simulink model "grid_connected_inverter_model"  (R2021a)
settings: Solver=VariableStepAuto  StartTime=0.0  StopTime=0.2  RelTol=1e-3
values from neighbouring files (symbols this model uses):
  I = 0    [grid_connected_inverter_tuning.m]
  I_max = A_inv/V_dc    (= 72.4637681159)    [grid_connected_inverter_tuning.m]
  Ki_current = alpha_current*R    [grid_connected_inverter_tuning.m]
  Ki_DC_voltage = Kp_DC_voltage/Ti_DC_voltage    [grid_connected_inverter_tuning.m]
  Ki_PLL = Kp_PLL/Ti_PLL    (= 21.16)    [grid_connected_inverter_tuning.m]
  Kp_current = alpha_current*L    [grid_connected_inverter_tuning.m]
  Kp_DC_voltage = 1    [grid_connected_inverter_tuning.m]
  Kp_PLL = 9.2/settling_time    (= 9.2)    [grid_connected_inverter_tuning.m]
  L = 1e-3    (= 0.001)    [grid_connected_inverter_tuning.m]
  omega = 2*pi*50    (= 314.159265359)    [grid_connected_inverter_tuning.m]
  R = 0.314    [grid_connected_inverter_tuning.m]
  sampling_time = 1/(2*switching_frequency)    (= 0.0002)    [grid_connected_inverter_tuning.m]
  V_a = 400    [grid_connected_inverter_tuning.m]
  V_b = 400    [grid_connected_inverter_tuning.m]
  V_c = 400    [grid_connected_inverter_tuning.m]
  V_dc = 690    [grid_connected_inverter_tuning.m]
libraries: fl_lib x17, ee_lib x15, nesl_utility x15, spsAlphaBetaZerotodq0Lib x6, pid_lib x5, spsabctoAlphaBetaZeroLib x4, spsAlphaBetaZerotoabcLib x1, spsdq0toAlphaBetaZeroLib x1, spsPWMGenerator2LevelLib x1
settings Model: SimulationMode=accelerator  Creator=giuli  LastModifiedBy=giuli
settings ModelReferenceCC: ModelReferenceMinAlgLoopOccurrences=on

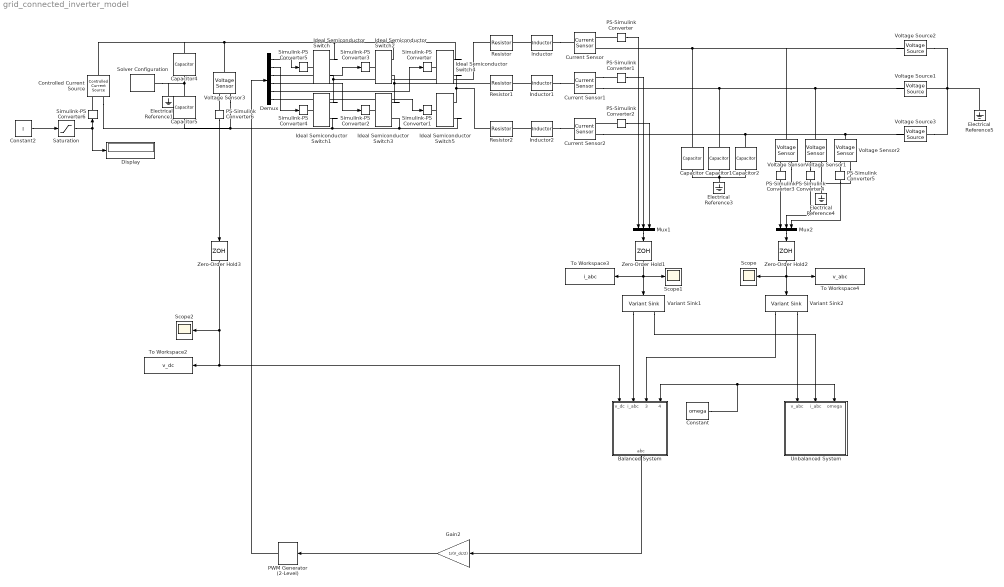
== system grid_connected_inverter_model ==
  Balanced System : Subsystem
  Capacitor : fl_lib/Electrical/Electrical Elements/Capacitor  c=C F  r=1e-6 Ohm  g=0 1/Ohm  i_specify=off  i_priority=None  i=0 A  i_nominal_specify=off  i_nominal_unit=A  i_nominal_value=1  v_specify=off  v_priority=None  v=0 V  v_nominal_specify=off  v_nominal_unit=V  v_nominal_value=1  vc_specify=off  vc_priority=High  vc=0 V  vc_nominal_specify=off  vc_nominal_unit=V  vc_nominal_value=1
  Capacitor1 : fl_lib/Electrical/Electrical Elements/Capacitor  c=C F  r=1e-6 Ohm  g=0 1/Ohm  i_specify=off  i_priority=None  i=0 A  i_nominal_specify=off  i_nominal_unit=A  i_nominal_value=1  v_specify=off  v_priority=None  v=0 V  v_nominal_specify=off  v_nominal_unit=V  v_nominal_value=1  vc_specify=off  vc_priority=High  vc=0 V  vc_nominal_specify=off  vc_nominal_unit=V  vc_nominal_value=1
  Capacitor2 : fl_lib/Electrical/Electrical Elements/Capacitor  c=C F  r=1e-6 Ohm  g=0 1/Ohm  i_specify=off  i_priority=None  i=0 A  i_nominal_specify=off  i_nominal_unit=A  i_nominal_value=1  v_specify=off  v_priority=None  v=0 V  v_nominal_specify=off  v_nominal_unit=V  v_nominal_value=1  vc_specify=off  vc_priority=High  vc=0 V  vc_nominal_specify=off  vc_nominal_unit=V  vc_nominal_value=1
  Capacitor4 : fl_lib/Electrical/Electrical Elements/Capacitor  c=C_dc F  r=1e-6 Ohm  g=0 1/Ohm  i_specify=off  i_priority=High  i=0 A  i_nominal_specify=off  i_nominal_unit=A  i_nominal_value=1  v_specify=off  v_priority=High  v=V_dc/2 V  v_nominal_specify=off  v_nominal_unit=V  v_nominal_value=1  vc_specify=on  vc_priority=High  vc=V_dc/2 V  vc_nominal_specify=off  vc_nominal_unit=V  vc_nominal_value=1
  Capacitor5 : fl_lib/Electrical/Electrical Elements/Capacitor  c=C_dc F  r=1e-6 Ohm  g=0 1/Ohm  i_specify=off  i_priority=High  i=0 A  i_nominal_specify=off  i_nominal_unit=A  i_nominal_value=1  v_specify=off  v_priority=High  v=V_dc/2 V  v_nominal_specify=off  v_nominal_unit=V  v_nominal_value=1  vc_specify=on  vc_priority=High  vc=V_dc/2 V  vc_nominal_specify=off  vc_nominal_unit=V  vc_nominal_value=1
  Constant : Constant  Value=omega
  Constant2 : Constant  Value=I
  Controlled Current Source : fl_lib/Electrical/Electrical Sources/Controlled Current Source
  Current Sensor : fl_lib/Electrical/Electrical Sensors/Current Sensor
  Current Sensor1 : fl_lib/Electrical/Electrical Sensors/Current Sensor
  Current Sensor2 : fl_lib/Electrical/Electrical Sensors/Current Sensor
  Demux : Demux  Outputs=6
  Display : Display
  Electrical Reference{1,3..5} (4 alike) : fl_lib/Electrical/Electrical Elements/Electrical Reference
  Gain2 : Gain  Gain=1/(V_dc/2)
  Ideal Semiconductor Switch{,1..5} (6 alike) : ee_lib/Semiconductors & Converters/Ideal Semiconductor Switch  Ron=0.001 Ohm  Goff=1e-6 1/Ohm  Vth=0.5 V  diode_param=1  diode_Vf=0.8 V  diode_Ron=0.001 Ohm  diode_Goff=1e-5 1/Ohm  diode_C=50e-9 F  diode_iRM=-235 A  diode_iF=300 A  diode_idot=-50 A/us  diode_trr_param=1  diode_trr_factor=3  diode_trr=15 us  diode_Qrr=1500 s*uA
      settings: SourceProductBaseCode=PS
  Inductor : ee_lib/Passive/Inductor  l=L H  L_tol=20  enable_L_tol=0  tol_distribution=1  nSigma=4  r=0 Ohm  g=1e-9 1/Ohm  enable_operating_limits=0  operating_limit_action=2  max_working_current=1 A  power_rating=1 W  enable_faults=0  fault_action=1  lambdaPercent=50  k_faulted=0.9999  turnsShort=0  openCct=0  groundShort=0  groundShortG=0 1/Ohm  tau_fault=1e-3 s  enable_temporal_fault=0  t_fault=1 s  enable_behavioral_fault=0  max_permissible_voltage=100 V  n_fail_on_voltage=1  max_permissible_current=1 A  t_fail_on_current=1 s  i_L_specify=off  i_L_priority=High  i_L=0 A  i_L_nominal_specify=off  i_L_nominal_unit=A  i_L_nominal_value=1
  Inductor1 : ee_lib/Passive/Inductor  l=L H  L_tol=20  enable_L_tol=0  tol_distribution=1  nSigma=4  r=0 Ohm  g=1e-9 1/Ohm  enable_operating_limits=0  operating_limit_action=2  max_working_current=1 A  power_rating=1 W  enable_faults=0  fault_action=1  lambdaPercent=50  k_faulted=0.9999  turnsShort=0  openCct=0  groundShort=0  groundShortG=0 1/Ohm  tau_fault=1e-3 s  enable_temporal_fault=0  t_fault=1 s  enable_behavioral_fault=0  max_permissible_voltage=100 V  n_fail_on_voltage=1  max_permissible_current=1 A  t_fail_on_current=1 s  i_L_specify=off  i_L_priority=High  i_L=0 A  i_L_nominal_specify=off  i_L_nominal_unit=A  i_L_nominal_value=1
  Inductor2 : ee_lib/Passive/Inductor  l=L H  L_tol=20  enable_L_tol=0  tol_distribution=1  nSigma=4  r=0 Ohm  g=1e-9 1/Ohm  enable_operating_limits=0  operating_limit_action=2  max_working_current=1 A  power_rating=1 W  enable_faults=0  fault_action=1  lambdaPercent=50  k_faulted=0.9999  turnsShort=0  openCct=0  groundShort=0  groundShortG=0 1/Ohm  tau_fault=1e-3 s  enable_temporal_fault=0  t_fault=1 s  enable_behavioral_fault=0  max_permissible_voltage=100 V  n_fail_on_voltage=1  max_permissible_current=1 A  t_fail_on_current=1 s  i_L_specify=off  i_L_priority=High  i_L=0 A  i_L_nominal_specify=off  i_L_nominal_unit=A  i_L_nominal_value=1
  Mux1 : Mux  Inputs=3
  Mux2 : Mux  Inputs=3
  PS-Simulink Converter{,1..6} (7 alike) : nesl_utility/PS-Simulink Converter  PhysicalDomain=network_engine_domain  SubClassName=ps_output  LeftPortType=input  RightPortType=output  PseudoPeriodic=off  Frequencies=[]  Unit=inherit  AffineConversion=off
      settings: SourceProductBaseCode=PW,SS
  PWM Generator (2-Level) : spsPWMGenerator2LevelLib/PWM Generator (2-Level)  ModulatorType=Three-phase bridge (6 pulses)  ModulatorMode=Unsynchronized  Fc=switching_frequency  Pc=0  nF=27  MinMax="[ -1  1 ]"  SamplingTechnique=Asymmetrical regular (double edge)  ModulatingSignals=off  m=0.8  Freq=60  Phase=0  Ts=1e-6  ShowCarrierOutport=off
  Resistor : ee_lib/Passive/Resistor  R=R Ohm  R_tol=5  enable_R_tol=0  tol_distribution=1  nSigma=4  enable_operating_limits=0  operating_limit_action=2  max_working_voltage=100 V  power_rating=1 W  enable_faults=0  fault_action=1  R_faulted=inf Ohm  enable_temporal_fault=0  t_fault=1 s  enable_behavioral_fault=0  max_permissible_current=1 A  t_fail_on_current=1 s  noise_mode=0  sample_time=1e-3 s  repeatability=1  auto_seed=3499211588  user_seed=0  Tdevice=25 degC  alpha=3.93e-3 1/K  Tmeas=25 degC  thermal_mass=100 J/K  power_derating_T1=70 degC  power_derating_T2=155 degC  operating_temperature_range_vec=[-50, 150] degC  temperature_specify=off  temperature_priority=High  temperature=298.15 K  temperature_nominal_specify=off  temperature_nominal_unit=K  temperature_nominal_value=1
  Resistor1 : ee_lib/Passive/Resistor  R=R Ohm  R_tol=5  enable_R_tol=0  tol_distribution=1  nSigma=4  enable_operating_limits=0  operating_limit_action=2  max_working_voltage=100 V  power_rating=1 W  enable_faults=0  fault_action=1  R_faulted=inf Ohm  enable_temporal_fault=0  t_fault=1 s  enable_behavioral_fault=0  max_permissible_current=1 A  t_fail_on_current=1 s  noise_mode=0  sample_time=1e-3 s  repeatability=1  auto_seed=3890346746  user_seed=0  Tdevice=25 degC  alpha=3.93e-3 1/K  Tmeas=25 degC  thermal_mass=100 J/K  power_derating_T1=70 degC  power_derating_T2=155 degC  operating_temperature_range_vec=[-50, 150] degC  temperature_specify=off  temperature_priority=High  temperature=298.15 K  temperature_nominal_specify=off  temperature_nominal_unit=K  temperature_nominal_value=1
  Resistor2 : ee_lib/Passive/Resistor  R=R Ohm  R_tol=5  enable_R_tol=0  tol_distribution=1  nSigma=4  enable_operating_limits=0  operating_limit_action=2  max_working_voltage=100 V  power_rating=1 W  enable_faults=0  fault_action=1  R_faulted=inf Ohm  enable_temporal_fault=0  t_fault=1 s  enable_behavioral_fault=0  max_permissible_current=1 A  t_fail_on_current=1 s  noise_mode=0  sample_time=1e-3 s  repeatability=1  auto_seed=545404223  user_seed=0  Tdevice=25 degC  alpha=3.93e-3 1/K  Tmeas=25 degC  thermal_mass=100 J/K  power_derating_T1=70 degC  power_derating_T2=155 degC  operating_temperature_range_vec=[-50, 150] degC  temperature_specify=off  temperature_priority=High  temperature=298.15 K  temperature_nominal_specify=off  temperature_nominal_unit=K  temperature_nominal_value=1
  Saturation : Saturate  UpperLimit=I_max  LowerLimit=0
  Scope : Scope
  Scope1 : Scope
  Scope2 : Scope
  Simulink-PS Converter{,1..6} (7 alike) : nesl_utility/Simulink-PS Converter  PhysicalDomain=network_engine_domain  SubClassName=ps_input  LeftPortType=input  RightPortType=output  PseudoPeriodic=off  Frequencies=[]  NoiseDistribution=none  NoiseParameters=[]  Unit=1  AffineConversion=off  FilteringAndDerivatives=provide  SimscapeFilterOrder=1  InputFilterTimeConstant=0.001  UdotUserProvided=0
      settings: SourceProductBaseCode=PW,SS
  Solver Configuration : nesl_utility/Solver Configuration  PhysicalDomain=network_engine_domain  SubClassName=solver  LeftPortType=input  RightPortType=generic  Tones=[]  Harmonics=[]  SimulateNoise=off  Profile=off  UseLocalSampling=off  EnableSwitchedLinearOptims=on  FrequencyDomain=off  UseCCode=off  RelTol=0.001  AbsTol=1e-06  MinStep=1e-09  ToWorkspace=off  RevertToSquareIcSolve=off  NumHomotopyIterations=100  PhasorMode=off  PhasorModeNumHarmonics=1  DoDC=off  ResidualTolerance=1e-09  UseLocalSolver=off  LocalSolverChoice=NE_BACKWARD_EULER_ADVANCER  LocalSolverSampleTime=0.001  DoFixedCost=off  MaxNonlinIter=3  MaxModeIter=2  ComputeImpulses=off  ImpulseIterations=2  LinearAlgebra=auto  EquationFormulation=NE_TIME_EF  DelaysMemoryBudget=1024  AutomaticFiltering=on  FilteringTimeConstant=0.001  PartitionStorageMethod=AS_NEEDED  PartitionMemoryBudget=1024  PartitionMethod=ROBUST
      settings: SourceProductBaseCode=PW,SS
  To Workspace2 : ToWorkspace  VariableName=v_dc  SaveFormat=Timeseries  SampleTime=-1
  To Workspace3 : ToWorkspace  VariableName=i_abc  SaveFormat=Timeseries  SampleTime=-1
  To Workspace4 : ToWorkspace  VariableName=v_abc  SaveFormat=Timeseries  SampleTime=-1
  Unbalanced System : Subsystem
  Variant Sink1 : VariantSink
  Variant Sink2 : VariantSink
  Voltage Sensor{,1..3} (4 alike) : fl_lib/Electrical/Electrical Sensors/Voltage Sensor
  Voltage Source1 : ee_lib/Sources/Voltage Source  dc_voltage=0 V  ac_voltage=V_b*sqrt(2)/sqrt(3) V  ac_shift=phi_b rad  ac_frequency=50 Hz  noise_mode=0  PSD=0 V^2/Hz  repeatability=1  auto_seed=1127352614  user_seed=0  sample_time=1e-3 s  i_specify=off  i_priority=None  i=0 A  i_nominal_specify=off  i_nominal_unit=A  i_nominal_value=1  v_specify=off  v_priority=None  v=0 V  v_nominal_specify=off  v_nominal_unit=V  v_nominal_value=1
  Voltage Source2 : ee_lib/Sources/Voltage Source  dc_voltage=0 V  ac_voltage=V_a*sqrt(2)/sqrt(3) V  ac_shift=phi_a rad  ac_frequency=50 Hz  noise_mode=0  PSD=0 V^2/Hz  repeatability=1  auto_seed=3440331608  user_seed=0  sample_time=1e-3 s  i_specify=off  i_priority=None  i=0 A  i_nominal_specify=off  i_nominal_unit=A  i_nominal_value=1  v_specify=off  v_priority=None  v=0 V  v_nominal_specify=off  v_nominal_unit=V  v_nominal_value=1
  Voltage Source3 : ee_lib/Sources/Voltage Source  dc_voltage=0 V  ac_voltage=V_c*sqrt(2)/sqrt(3) V  ac_shift=phi_c rad  ac_frequency=50 Hz  noise_mode=0  PSD=0 V^2/Hz  repeatability=1  auto_seed=830791639  user_seed=0  sample_time=1e-3 s  i_specify=off  i_priority=None  i=0 A  i_nominal_specify=off  i_nominal_unit=A  i_nominal_value=1  v_specify=off  v_priority=None  v=0 V  v_nominal_specify=off  v_nominal_unit=V  v_nominal_value=1
  Zero-Order Hold1 : ZeroOrderHold  SampleTime=sampling_time
  Zero-Order Hold2 : ZeroOrderHold  SampleTime=sampling_time
  Zero-Order Hold3 : ZeroOrderHold  SampleTime=sampling_time
  wires:
  PS-Simulink Converter/1 -> Mux1/1
  PS-Simulink Converter1/1 -> Mux1/2
  PS-Simulink Converter2/1 -> Mux1/3
  PS-Simulink Converter4/1 -> Mux2/2
  PS-Simulink Converter5/1 -> Mux2/3
  PWM Generator (2-Level)/1 -> Demux/1
  Mux1/1 -> Zero-Order Hold1/1
  PS-Simulink Converter3/1 -> Mux2/1
  Mux2/1 -> Zero-Order Hold2/1
  Zero-Order Hold2/1 -> Scope/1, Variant Sink2/1, To Workspace4/1
  Gain2/1 -> PWM Generator (2-Level)/1
  Demux/1 -> Simulink-PS Converter5/1
  Demux/2 -> Simulink-PS Converter4/1
  Demux/3 -> Simulink-PS Converter3/1
  Demux/4 -> Simulink-PS Converter2/1
  Demux/5 -> Simulink-PS Converter/1
  Demux/6 -> Simulink-PS Converter1/1
  PS-Simulink Converter6/1 -> Zero-Order Hold3/1
  Constant/1 -> Balanced System/4(omega), Unbalanced System/3(omega)
  Zero-Order Hold3/1 -> Scope2/1, Balanced System/1(v_dc), To Workspace2/1
  Variant Sink1/1 -> Balanced System/2(i_abc)
  Variant Sink1/2 -> Unbalanced System/2(i_abc)
  Variant Sink2/2 -> Unbalanced System/1(v_abc)
  Balanced System/1(abc) -> Gain2/1
  Variant Sink2/1 -> Balanced System/3(v_abc)
  Constant2/1 -> Saturation/1
  Saturation/1 -> Simulink-PS Converter6/1, Display/1
  Zero-Order Hold1/1 -> To Workspace3/1, Scope1/1, Variant Sink1/1
  connections:
  Simulink-PS Converter/RConn1 -- Ideal Semiconductor Switch4/LConn1
  Simulink-PS Converter1/RConn1 -- Ideal Semiconductor Switch5/LConn1
  Simulink-PS Converter2/RConn1 -- Ideal Semiconductor Switch3/LConn1
  Simulink-PS Converter3/RConn1 -- Ideal Semiconductor Switch2/LConn1
  Simulink-PS Converter4/RConn1 -- Ideal Semiconductor Switch1/LConn1
  Simulink-PS Converter5/RConn1 -- Ideal Semiconductor Switch/LConn1
  Ideal Semiconductor Switch/RConn1 -- Capacitor4/LConn1 -- Controlled Current Source/LConn1 -- Voltage Sensor3/LConn1 -- Ideal Semiconductor Switch4/RConn1 -- Ideal Semiconductor Switch2/RConn1
  Ideal Semiconductor Switch1/RConn1 -- Resistor/LConn1 -- Ideal Semiconductor Switch/RConn2
  Ideal Semiconductor Switch1/RConn2 -- Controlled Current Source/RConn2 -- Capacitor5/RConn1 -- Voltage Sensor3/RConn2 -- Ideal Semiconductor Switch5/RConn2 -- Ideal Semiconductor Switch3/RConn2
  Ideal Semiconductor Switch3/RConn1 -- Resistor1/LConn1 -- Ideal Semiconductor Switch2/RConn2
  Ideal Semiconductor Switch4/RConn2 -- Ideal Semiconductor Switch5/RConn1 -- Resistor2/LConn1
  Current Sensor1/RConn2 -- Capacitor1/LConn1 -- Voltage Source1/LConn1 -- Voltage Sensor1/LConn1
  PS-Simulink Converter3/LConn1 -- Voltage Sensor/RConn1
  PS-Simulink Converter5/LConn1 -- Voltage Sensor2/RConn1
  Voltage Sensor1/RConn1 -- PS-Simulink Converter4/LConn1
  Current Sensor2/RConn2 -- Capacitor2/LConn1 -- Voltage Source3/LConn1 -- Voltage Sensor2/LConn1
  Capacitor/LConn1 -- Voltage Source2/LConn1 -- Voltage Sensor/LConn1 -- Current Sensor/RConn2
  Capacitor/RConn1 -- Electrical Reference3/LConn1 -- Capacitor2/RConn1 -- Capacitor1/RConn1
  Voltage Sensor/RConn2 -- Electrical Reference4/LConn1 -- Voltage Sensor2/RConn2 -- Voltage Sensor1/RConn2
  PS-Simulink Converter/LConn1 -- Current Sensor/RConn1
  Inductor1/RConn1 -- Current Sensor1/LConn1
  PS-Simulink Converter2/LConn1 -- Current Sensor2/RConn1
  Inductor2/RConn1 -- Current Sensor2/LConn1
  Inductor/RConn1 -- Current Sensor/LConn1
  Current Sensor1/RConn1 -- PS-Simulink Converter1/LConn1
  Inductor/LConn1 -- Resistor/RConn1
  Inductor1/LConn1 -- Resistor1/RConn1
  Inductor2/LConn1 -- Resistor2/RConn1
  PS-Simulink Converter6/LConn1 -- Voltage Sensor3/RConn1
  Simulink-PS Converter6/RConn1 -- Controlled Current Source/RConn1
  Capacitor4/RConn1 -- Solver Configuration/RConn1 -- Electrical Reference1/LConn1 -- Capacitor5/LConn1
  Electrical Reference5/LConn1 -- Voltage Source3/RConn1 -- Voltage Source2/RConn1 -- Voltage Source1/RConn1

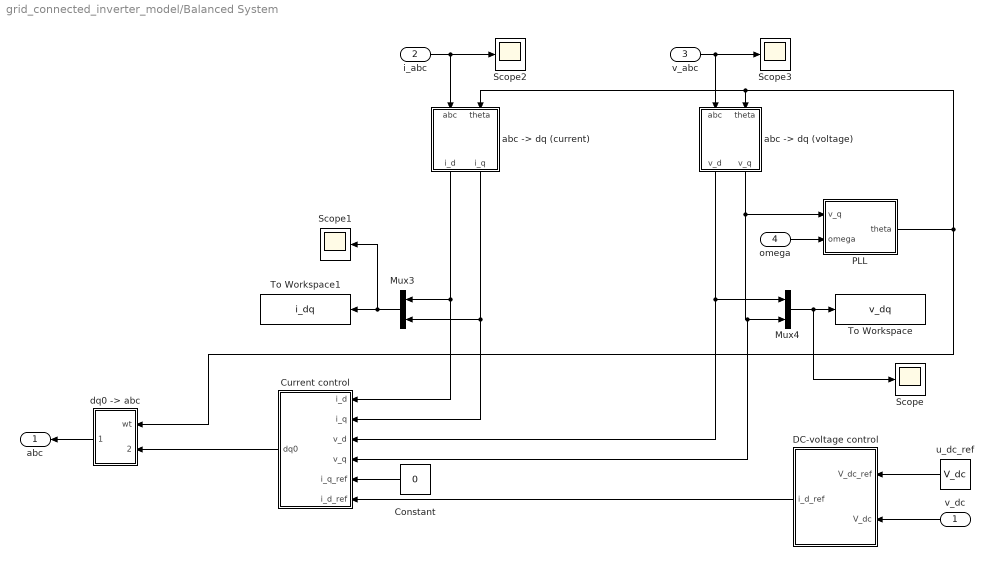
== system grid_connected_inverter_model/Balanced System ==
  v_dc : Inport
  i_abc : Inport  Port=2
  v_abc : Inport  Port=3
  omega : Inport  Port=4
  Constant : Constant  Value=0
  Current control : Subsystem  mask{kp_mask=Kp_current, ki_mask=Ki_current}
      mask prompts: kp_mask "kp"; ki_mask "ki"
      mask DialogControl ParameterGroupVar Prompt: Control Parameters
  DC-voltage control : Subsystem  mask{kp_mask=Kp_DC_voltage, ki_mask=Ki_DC_voltage}
      mask prompts: kp_mask "kp"; ki_mask "ki"
      mask DialogControl ParameterGroupVar Prompt: Control Parameters
  Mux3 : Mux  Inputs=2
  Mux4 : Mux  Inputs=2
  PLL : Subsystem  mask{kp_mask=Kp_PLL, ki_mask=Ki_PLL}
      mask prompts: kp_mask "kp"; ki_mask "ki"
  Scope{,1..3} (4 alike) : Scope
  To Workspace : ToWorkspace  VariableName=v_dq  SaveFormat=Timeseries  SampleTime=-1
  To Workspace1 : ToWorkspace  VariableName=i_dq  SaveFormat=Timeseries  SampleTime=-1
  "abc -> dq (current)" : Subsystem  TreatAsAtomicUnit=on
      settings: MinAlgLoopOccurrences=on
  "abc -> dq (voltage)" : Subsystem  TreatAsAtomicUnit=on
      settings: MinAlgLoopOccurrences=on
  "dq0 -> abc" : Subsystem  TreatAsAtomicUnit=on
      settings: MinAlgLoopOccurrences=on
  u_dc_ref : Constant  Value=V_dc
  abc : Outport
  wires:
  "abc -> dq (current)"/2(i_q) -> Current control/2(i_q), Mux3/2
  "abc -> dq (current)"/1(i_d) -> Current control/1(i_d), Mux3/1
  v_abc/1 -> Scope3/1, "abc -> dq (voltage)"/1(abc)
  v_dc/1 -> DC-voltage control/2(V_dc)
  "abc -> dq (voltage)"/2(v_q) -> Current control/4(v_q), Mux4/2, PLL/1(v_q)
  Current control/1(dq0) -> "dq0 -> abc"/2(dq0)
  PLL/1(theta) -> "abc -> dq (voltage)"/2(theta), "abc -> dq (current)"/2(theta), "dq0 -> abc"/1(wt)
  "abc -> dq (voltage)"/1(v_d) -> Mux4/1, Current control/3(v_d)
  u_dc_ref/1 -> DC-voltage control/1(V_dc_ref)
  Mux3/1 -> Scope1/1, To Workspace1/1
  Mux4/1 -> Scope/1, To Workspace/1
  DC-voltage control/1(i_d_ref) -> Current control/6(i_d_ref)
  i_abc/1 -> Scope2/1, "abc -> dq (current)"/1(abc)
  "dq0 -> abc"/1(abc) -> abc/1
  Constant/1 -> Current control/5(i_q_ref)
  omega/1 -> PLL/2(omega)

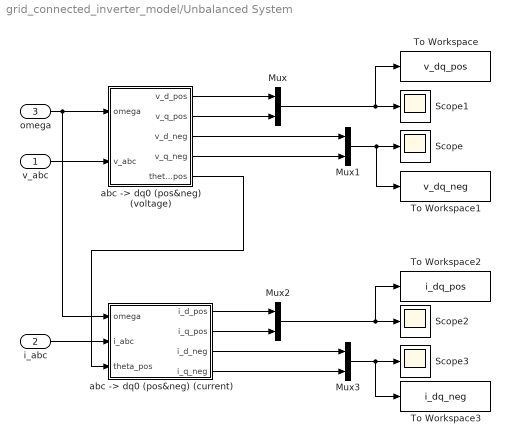
== system grid_connected_inverter_model/Unbalanced System ==
  v_abc : Inport
  i_abc : Inport  Port=2
  omega : Inport  Port=3
  Mux{,1..3} (4 alike) : Mux  Inputs=2
  Scope{,1..3} (4 alike) : Scope
  To Workspace : ToWorkspace  VariableName=v_dq_pos  SaveFormat=Timeseries  SampleTime=-1
  To Workspace1 : ToWorkspace  VariableName=v_dq_neg  SaveFormat=Timeseries  SampleTime=-1
  To Workspace2 : ToWorkspace  VariableName=i_dq_pos  SaveFormat=Timeseries  SampleTime=-1
  To Workspace3 : ToWorkspace  VariableName=i_dq_neg  SaveFormat=Timeseries  SampleTime=-1
  "abc -> dq0 (pos&neg) (current)" : Subsystem
  "abc -> dq0 (pos&neg) (voltage)" : Subsystem
  wires:
  v_abc/1 -> "abc -> dq0 (pos&neg) (voltage)"/2(v_abc)
  i_abc/1 -> "abc -> dq0 (pos&neg) (current)"/2(i_abc)
  "abc -> dq0 (pos&neg) (current)"/1(i_d_pos) -> Mux2/1
  "abc -> dq0 (pos&neg) (current)"/2(i_q_pos) -> Mux2/2
  "abc -> dq0 (pos&neg) (voltage)"/1(v_d_pos) -> Mux/1
  "abc -> dq0 (pos&neg) (voltage)"/2(v_q_pos) -> Mux/2
  "abc -> dq0 (pos&neg) (current)"/3(i_d_neg) -> Mux3/1
  "abc -> dq0 (pos&neg) (current)"/4(i_q_neg) -> Mux3/2
  "abc -> dq0 (pos&neg) (voltage)"/3(v_d_neg) -> Mux1/1
  "abc -> dq0 (pos&neg) (voltage)"/4(v_q_neg) -> Mux1/2
  omega/1 -> "abc -> dq0 (pos&neg) (current)"/1(omega), "abc -> dq0 (pos&neg) (voltage)"/1(omega)
  "abc -> dq0 (pos&neg) (voltage)"/5(theta_pos) -> "abc -> dq0 (pos&neg) (current)"/3(theta_pos)
  Mux1/1 -> To Workspace1/1, Scope/1
  Mux/1 -> To Workspace/1, Scope1/1
  Mux2/1 -> To Workspace2/1, Scope2/1
  Mux3/1 -> To Workspace3/1, Scope3/1

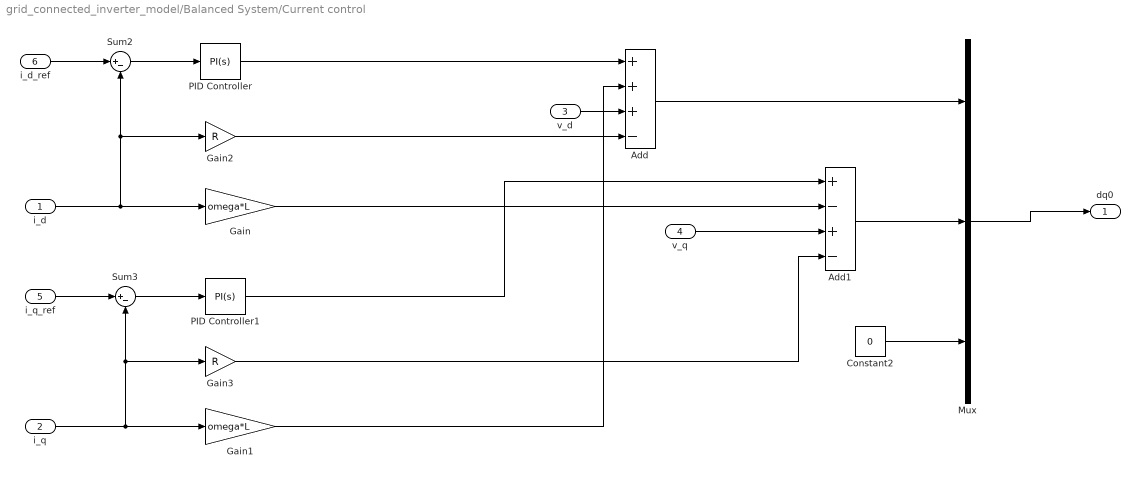
== system grid_connected_inverter_model/Balanced System/Current control ==
  i_d : Inport
  i_q : Inport  Port=2
  v_d : Inport  Port=3
  v_q : Inport  Port=4
  i_q_ref : Inport  Port=5
  i_d_ref : Inport  Port=6
  Add : Sum  Inputs=+++-
  Add1 : Sum  Inputs=+-+-
  Constant2 : Constant  Value=0
  Gain : Gain  Gain=omega*L
  Gain1 : Gain  Gain=omega*L
  Gain2 : Gain  Gain=R
  Gain3 : Gain  Gain=R
  Mux : Mux  Inputs=3
  PID Controller : pid_lib/PID Controller  Controller=PI  Form=Ideal  TimeDomain=Continuous-time  UseExternalTs=off  SampleTime=sampling_time  IntegratorMethod=Forward Euler  FilterMethod=Forward Euler  ControllerParametersSource=internal  P=kp_mask  I=ki_mask  D=0  UseFilter=on  N=100  TunerSelectOption=Transfer Function Based (PID Tuner App)  InitialConditionSource=internal  InitialConditionForIntegrator=0  InitialConditionForFilter=0  DifferentiatorICPrevScaledInput=0  ExternalReset=none  TrackingMode=off  Kt=1  LimitOutput=off  SatLimitsSource=internal  UpperSaturationLimit=inf  LowerSaturationLimit=-inf  LinearizeAsGain=on  AntiWindupMode=none  Kb=1  POutMin=[]  POutMax=[]  IOutMin=[]  IOutMax=[]  DOutMin=[]  DOutMax=[]  NOutMin=[]  NOutMax=[]  SumOutMin=[]  SumOutMax=[]  SaturationOutMin=[]  SaturationOutMax=[]  PParamMin=[]  PParamMax=[]  IParamMin=[]  IParamMax=[]  DParamMin=[]  DParamMax=[]  NParamMin=[]  NParamMax=[]  KbParamMin=[]  KbParamMax=[]  KtParamMin=[]  KtParamMax=[]  KbOutMin=[]  KbOutMax=[]  KtOutMin=[]  KtOutMax=[]  IntegratorOutMin=[]  IntegratorOutMax=[]  FilterOutMin=[]  FilterOutMax=[]  SumI1OutMin=[]  SumI1OutMax=[]  SumI2OutMin=[]  SumI2OutMax=[]  SumI3OutMin=[]  SumI3OutMax=[]  SumI4OutMin=[]  SumI4OutMax=[]  SumDOutMin=[]  SumDOutMax=[]  DifferentiatorOutMin=[]  DifferentiatorOutMax=[]  FilterDiffOutCoefMin=[]  FilterDiffOutCoefMax=[]  ReciprocalOutMin=[]  ReciprocalOutMax=[]  SumDenOutMin=[]  SumDenOutMax=[]  SumNumOutMin=[]  SumNumOutMax=[]  DivideOutMin=[]  DivideOutMax=[]  UdiffTsProdOutMin=[]  UdiffTsProdOutMax=[]  NTsProdOutMin=[]  NTsProdOutMax=[]  UintegralTsProdOutMin=[]  UintegralTsProdOutMax=[]  UngainTsProdOutMin=[]  UngainTsProdOutMax=[]  IntegratorContinuousStateAttributes=''  IntegratorStateMustResolveToSignalObject=off  IntegratorRTWStateStorageClass=Auto  FilterContinuousStateAttributes=''  FilterStateMustResolveToSignalObject=off  FilterRTWStateStorageClass=Auto  ParallelPVariant=Passthrough  IdealPVariant=InternalParameters  IVariant=InternalParameters  DVariant=Disabled  IntegratorVariant=Continuous  SatVariant=Disabled  AWVariant=Passthrough  PCopyVariant=Disabled  TRVariant=Disabled  FdbkBlocksVariant=Forward  IdealPFdbkVariant=Disabled  SatFdbkVariant=Disabled  DerivativeFilterVariant=Disabled  NVariant=Disabled  NCopyVariant=Disabled_SignalSpec  FilterICVariant=Disabled  IntegratorICVariant=InternalICs  ExternalResetVariant=Disabled  TRSumVariant=Passthrough  SumFdbkVariant=Disabled  SumVariant=Sum_PI  TsampFilterVariant=InternalTs  TsampNgainVariant=Passthrough  TsampIntegralVariant=Passthrough  ExternalSaturationOutDataTypeStr=Inherit: Same as second input
  PID Controller1 : pid_lib/PID Controller  Controller=PI  Form=Ideal  TimeDomain=Continuous-time  UseExternalTs=off  SampleTime=sampling_time  IntegratorMethod=Forward Euler  FilterMethod=Forward Euler  ControllerParametersSource=internal  P=kp_mask  I=ki_mask  D=0  UseFilter=on  N=100  TunerSelectOption=Transfer Function Based (PID Tuner App)  InitialConditionSource=internal  InitialConditionForIntegrator=0  InitialConditionForFilter=0  DifferentiatorICPrevScaledInput=0  ExternalReset=none  TrackingMode=off  Kt=1  LimitOutput=off  SatLimitsSource=internal  UpperSaturationLimit=inf  LowerSaturationLimit=-inf  LinearizeAsGain=on  AntiWindupMode=none  Kb=1  POutMin=[]  POutMax=[]  IOutMin=[]  IOutMax=[]  DOutMin=[]  DOutMax=[]  NOutMin=[]  NOutMax=[]  SumOutMin=[]  SumOutMax=[]  SaturationOutMin=[]  SaturationOutMax=[]  PParamMin=[]  PParamMax=[]  IParamMin=[]  IParamMax=[]  DParamMin=[]  DParamMax=[]  NParamMin=[]  NParamMax=[]  KbParamMin=[]  KbParamMax=[]  KtParamMin=[]  KtParamMax=[]  KbOutMin=[]  KbOutMax=[]  KtOutMin=[]  KtOutMax=[]  IntegratorOutMin=[]  IntegratorOutMax=[]  FilterOutMin=[]  FilterOutMax=[]  SumI1OutMin=[]  SumI1OutMax=[]  SumI2OutMin=[]  SumI2OutMax=[]  SumI3OutMin=[]  SumI3OutMax=[]  SumI4OutMin=[]  SumI4OutMax=[]  SumDOutMin=[]  SumDOutMax=[]  DifferentiatorOutMin=[]  DifferentiatorOutMax=[]  FilterDiffOutCoefMin=[]  FilterDiffOutCoefMax=[]  ReciprocalOutMin=[]  ReciprocalOutMax=[]  SumDenOutMin=[]  SumDenOutMax=[]  SumNumOutMin=[]  SumNumOutMax=[]  DivideOutMin=[]  DivideOutMax=[]  UdiffTsProdOutMin=[]  UdiffTsProdOutMax=[]  NTsProdOutMin=[]  NTsProdOutMax=[]  UintegralTsProdOutMin=[]  UintegralTsProdOutMax=[]  UngainTsProdOutMin=[]  UngainTsProdOutMax=[]  IntegratorContinuousStateAttributes=''  IntegratorStateMustResolveToSignalObject=off  IntegratorRTWStateStorageClass=Auto  FilterContinuousStateAttributes=''  FilterStateMustResolveToSignalObject=off  FilterRTWStateStorageClass=Auto  ParallelPVariant=Passthrough  IdealPVariant=InternalParameters  IVariant=InternalParameters  DVariant=Disabled  IntegratorVariant=Continuous  SatVariant=Disabled  AWVariant=Passthrough  PCopyVariant=Disabled  TRVariant=Disabled  FdbkBlocksVariant=Forward  IdealPFdbkVariant=Disabled  SatFdbkVariant=Disabled  DerivativeFilterVariant=Disabled  NVariant=Disabled  NCopyVariant=Disabled_SignalSpec  FilterICVariant=Disabled  IntegratorICVariant=InternalICs  ExternalResetVariant=Disabled  TRSumVariant=Passthrough  SumFdbkVariant=Disabled  SumVariant=Sum_PI  TsampFilterVariant=InternalTs  TsampNgainVariant=Passthrough  TsampIntegralVariant=Passthrough  ExternalSaturationOutDataTypeStr=Inherit: Same as second input
  Sum2 : Sum  Inputs=|+-
  Sum3 : Sum  Inputs=|+-
  dq0 : Outport
  wires:
  Add1/1 -> Mux/2
  Add/1 -> Mux/1
  Constant2/1 -> Mux/3
  PID Controller/1 -> Add/1
  Gain/1 -> Add1/2
  Gain1/1 -> Add/2
  Sum2/1 -> PID Controller/1
  Mux/1 -> dq0/1
  v_d/1 -> Add/3
  Sum3/1 -> PID Controller1/1
  i_q/1 -> Gain3/1, Sum3/2, Gain1/1
  i_d/1 -> Gain/1, Sum2/2, Gain2/1
  PID Controller1/1 -> Add1/1
  i_d_ref/1 -> Sum2/1
  i_q_ref/1 -> Sum3/1
  v_q/1 -> Add1/3
  Gain2/1 -> Add/4
  Gain3/1 -> Add1/4

== system grid_connected_inverter_model/Balanced System/DC-voltage control ==
  V_dc_ref : Inport
  V_dc : Inport  Port=2
  PID Controller3 : pid_lib/PID Controller  Controller=PI  Form=Ideal  TimeDomain=Continuous-time  UseExternalTs=off  SampleTime=-1  IntegratorMethod=Forward Euler  FilterMethod=Forward Euler  ControllerParametersSource=internal  P=kp_mask  I=ki_mask  D=0  UseFilter=on  N=100  TunerSelectOption=Transfer Function Based (PID Tuner App)  InitialConditionSource=internal  InitialConditionForIntegrator=0  InitialConditionForFilter=0  DifferentiatorICPrevScaledInput=0  ExternalReset=none  TrackingMode=off  Kt=1  LimitOutput=off  SatLimitsSource=internal  UpperSaturationLimit=inf  LowerSaturationLimit=-inf  LinearizeAsGain=on  AntiWindupMode=none  Kb=1  POutMin=[]  POutMax=[]  IOutMin=[]  IOutMax=[]  DOutMin=[]  DOutMax=[]  NOutMin=[]  NOutMax=[]  SumOutMin=[]  SumOutMax=[]  SaturationOutMin=[]  SaturationOutMax=[]  PParamMin=[]  PParamMax=[]  IParamMin=[]  IParamMax=[]  DParamMin=[]  DParamMax=[]  NParamMin=[]  NParamMax=[]  KbParamMin=[]  KbParamMax=[]  KtParamMin=[]  KtParamMax=[]  KbOutMin=[]  KbOutMax=[]  KtOutMin=[]  KtOutMax=[]  IntegratorOutMin=[]  IntegratorOutMax=[]  FilterOutMin=[]  FilterOutMax=[]  SumI1OutMin=[]  SumI1OutMax=[]  SumI2OutMin=[]  SumI2OutMax=[]  SumI3OutMin=[]  SumI3OutMax=[]  SumI4OutMin=[]  SumI4OutMax=[]  SumDOutMin=[]  SumDOutMax=[]  DifferentiatorOutMin=[]  DifferentiatorOutMax=[]  FilterDiffOutCoefMin=[]  FilterDiffOutCoefMax=[]  ReciprocalOutMin=[]  ReciprocalOutMax=[]  SumDenOutMin=[]  SumDenOutMax=[]  SumNumOutMin=[]  SumNumOutMax=[]  DivideOutMin=[]  DivideOutMax=[]  UdiffTsProdOutMin=[]  UdiffTsProdOutMax=[]  NTsProdOutMin=[]  NTsProdOutMax=[]  UintegralTsProdOutMin=[]  UintegralTsProdOutMax=[]  UngainTsProdOutMin=[]  UngainTsProdOutMax=[]  IntegratorContinuousStateAttributes=''  IntegratorStateMustResolveToSignalObject=off  IntegratorRTWStateStorageClass=Auto  FilterContinuousStateAttributes=''  FilterStateMustResolveToSignalObject=off  FilterRTWStateStorageClass=Auto  ParallelPVariant=Passthrough  IdealPVariant=InternalParameters  IVariant=InternalParameters  DVariant=Disabled  IntegratorVariant=Continuous  SatVariant=Disabled  AWVariant=Passthrough  PCopyVariant=Disabled  TRVariant=Disabled  FdbkBlocksVariant=Forward  IdealPFdbkVariant=Disabled  SatFdbkVariant=Disabled  DerivativeFilterVariant=Disabled  NVariant=Disabled  NCopyVariant=Disabled_SignalSpec  FilterICVariant=Disabled  IntegratorICVariant=InternalICs  ExternalResetVariant=Disabled  TRSumVariant=Passthrough  SumFdbkVariant=Disabled  SumVariant=Sum_PI  TsampFilterVariant=InternalTs  TsampNgainVariant=Passthrough  TsampIntegralVariant=Passthrough  ExternalSaturationOutDataTypeStr=Inherit: Same as second input
  Sum6 : Sum  Inputs=|-+
  i_d_ref : Outport
  wires:
  Sum6/1 -> PID Controller3/1
  V_dc_ref/1 -> Sum6/1
  V_dc/1 -> Sum6/2
  PID Controller3/1 -> i_d_ref/1

== system grid_connected_inverter_model/Balanced System/PLL ==
  v_q : Inport
  omega : Inport  Port=2
  Gain : Gain
  Integrator : Integrator
  PID Controller : pid_lib/PID Controller  Controller=PI  Form=Ideal  TimeDomain=Continuous-time  UseExternalTs=off  SampleTime=-1  IntegratorMethod=Forward Euler  FilterMethod=Forward Euler  ControllerParametersSource=internal  P=kp_mask  I=ki_mask  D=0  UseFilter=on  N=100  TunerSelectOption=Transfer Function Based (PID Tuner App)  InitialConditionSource=internal  InitialConditionForIntegrator=0  InitialConditionForFilter=0  DifferentiatorICPrevScaledInput=0  ExternalReset=none  TrackingMode=off  Kt=1  LimitOutput=off  SatLimitsSource=internal  UpperSaturationLimit=inf  LowerSaturationLimit=-inf  LinearizeAsGain=on  AntiWindupMode=none  Kb=1  POutMin=[]  POutMax=[]  IOutMin=[]  IOutMax=[]  DOutMin=[]  DOutMax=[]  NOutMin=[]  NOutMax=[]  SumOutMin=[]  SumOutMax=[]  SaturationOutMin=[]  SaturationOutMax=[]  PParamMin=[]  PParamMax=[]  IParamMin=[]  IParamMax=[]  DParamMin=[]  DParamMax=[]  NParamMin=[]  NParamMax=[]  KbParamMin=[]  KbParamMax=[]  KtParamMin=[]  KtParamMax=[]  KbOutMin=[]  KbOutMax=[]  KtOutMin=[]  KtOutMax=[]  IntegratorOutMin=[]  IntegratorOutMax=[]  FilterOutMin=[]  FilterOutMax=[]  SumI1OutMin=[]  SumI1OutMax=[]  SumI2OutMin=[]  SumI2OutMax=[]  SumI3OutMin=[]  SumI3OutMax=[]  SumI4OutMin=[]  SumI4OutMax=[]  SumDOutMin=[]  SumDOutMax=[]  DifferentiatorOutMin=[]  DifferentiatorOutMax=[]  FilterDiffOutCoefMin=[]  FilterDiffOutCoefMax=[]  ReciprocalOutMin=[]  ReciprocalOutMax=[]  SumDenOutMin=[]  SumDenOutMax=[]  SumNumOutMin=[]  SumNumOutMax=[]  DivideOutMin=[]  DivideOutMax=[]  UdiffTsProdOutMin=[]  UdiffTsProdOutMax=[]  NTsProdOutMin=[]  NTsProdOutMax=[]  UintegralTsProdOutMin=[]  UintegralTsProdOutMax=[]  UngainTsProdOutMin=[]  UngainTsProdOutMax=[]  IntegratorContinuousStateAttributes=''  IntegratorStateMustResolveToSignalObject=off  IntegratorRTWStateStorageClass=Auto  FilterContinuousStateAttributes=''  FilterStateMustResolveToSignalObject=off  FilterRTWStateStorageClass=Auto  ParallelPVariant=Passthrough  IdealPVariant=InternalParameters  IVariant=InternalParameters  DVariant=Disabled  IntegratorVariant=Continuous  SatVariant=Disabled  AWVariant=Passthrough  PCopyVariant=Disabled  TRVariant=Disabled  FdbkBlocksVariant=Forward  IdealPFdbkVariant=Disabled  SatFdbkVariant=Disabled  DerivativeFilterVariant=Disabled  NVariant=Disabled  NCopyVariant=Disabled_SignalSpec  FilterICVariant=Disabled  IntegratorICVariant=InternalICs  ExternalResetVariant=Disabled  TRSumVariant=Passthrough  SumFdbkVariant=Disabled  SumVariant=Sum_PI  TsampFilterVariant=InternalTs  TsampNgainVariant=Passthrough  TsampIntegralVariant=Passthrough  ExternalSaturationOutDataTypeStr=Inherit: Same as second input
  Sum : Sum  Inputs=|++
  theta : Outport
  wires:
  v_q/1 -> PID Controller/1
  omega/1 -> Sum/2
  Integrator/1 -> theta/1
  PID Controller/1 -> Sum/1
  Sum/1 -> Gain/1
  Gain/1 -> Integrator/1

== system grid_connected_inverter_model/Balanced System/abc -> dq (current) ==
  abc : Inport
  theta : Inport  Port=2
  Alpha-Beta-Zero to dq0 : spsAlphaBetaZerotodq0Lib/Alpha-Beta-Zero to dq0  Alignment=Aligned with phase A axis
      settings: SourceProductBaseCode=PS
  Demux : Demux  Outputs=3
  Terminator : Terminator
  abc to Alpha-Beta-Zero1 : spsabctoAlphaBetaZeroLib/abc to Alpha-Beta-Zero
      settings: SourceProductBaseCode=PS
  i_d : Outport
  i_q : Outport  Port=2
  wires:
  Alpha-Beta-Zero to dq0/1 -> Demux/1
  Demux/3 -> Terminator/1
  Demux/1 -> i_d/1
  abc/1 -> abc to Alpha-Beta-Zero1/1
  Demux/2 -> i_q/1
  abc to Alpha-Beta-Zero1/1 -> Alpha-Beta-Zero to dq0/1
  theta/1 -> Alpha-Beta-Zero to dq0/2

== system grid_connected_inverter_model/Balanced System/abc -> dq (voltage) ==
  abc : Inport
  theta : Inport  Port=2
  Alpha-Beta-Zero to dq0 : spsAlphaBetaZerotodq0Lib/Alpha-Beta-Zero to dq0  Alignment=Aligned with phase A axis
      settings: SourceProductBaseCode=PS
  Demux3 : Demux  Outputs=3
  Terminator : Terminator
  abc to Alpha-Beta-Zero : spsabctoAlphaBetaZeroLib/abc to Alpha-Beta-Zero
      settings: SourceProductBaseCode=PS
  v_d : Outport
  v_q : Outport  Port=2
  wires:
  Demux3/2 -> v_q/1
  Demux3/1 -> v_d/1
  theta/1 -> Alpha-Beta-Zero to dq0/2
  Alpha-Beta-Zero to dq0/1 -> Demux3/1
  abc to Alpha-Beta-Zero/1 -> Alpha-Beta-Zero to dq0/1
  abc/1 -> abc to Alpha-Beta-Zero/1
  Demux3/3 -> Terminator/1

== system grid_connected_inverter_model/Balanced System/dq0 -> abc ==
  wt : Inport
  dq0 : Inport  Port=2
  Alpha-Beta-Zero to abc : spsAlphaBetaZerotoabcLib/Alpha-Beta-Zero to abc
      settings: SourceProductBaseCode=PS
  dq0 to Alpha-Beta-Zero : spsdq0toAlphaBetaZeroLib/dq0 to Alpha-Beta-Zero  Alignment=Aligned with phase A axis
      settings: SourceProductBaseCode=PS
  abc : Outport
  wires:
  dq0 to Alpha-Beta-Zero/1 -> Alpha-Beta-Zero to abc/1
  dq0/1 -> dq0 to Alpha-Beta-Zero/1
  wt/1 -> dq0 to Alpha-Beta-Zero/2
  Alpha-Beta-Zero to abc/1 -> abc/1

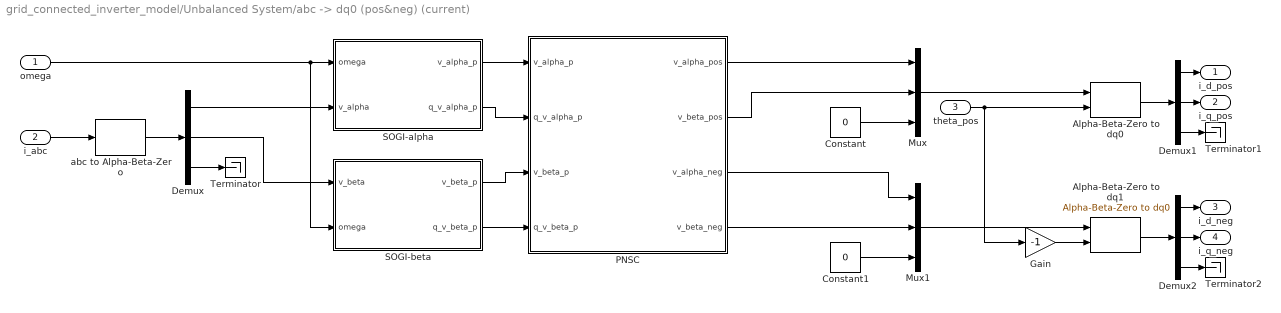
== system grid_connected_inverter_model/Unbalanced System/abc -> dq0 (pos&neg) (current) ==
  omega : Inport
  i_abc : Inport  Port=2
  theta_pos : Inport  Port=3
  Alpha-Beta-Zero to dq0 : spsAlphaBetaZerotodq0Lib/Alpha-Beta-Zero to dq0  Alignment=Aligned with phase A axis
      settings: SourceProductBaseCode=PS
  Alpha-Beta-Zero to dq1 : spsAlphaBetaZerotodq0Lib/Alpha-Beta-Zero to dq0  Alignment=Aligned with phase A axis
      settings: SourceProductBaseCode=PS
  Constant : Constant  Value=0
  Constant1 : Constant  Value=0
  Demux : Demux  Outputs=3
  Demux1 : Demux  Outputs=3
  Demux2 : Demux  Outputs=3
  Gain : Gain  Gain=-1
  Mux : Mux  Inputs=3
  Mux1 : Mux  Inputs=3
  PNSC : Subsystem
  SOGI-alpha : Subsystem  mask{t_s=0.01}
      mask prompts: t_s "Settling time [s]"
  SOGI-beta : Subsystem  mask{t_s=0.01}
      mask prompts: t_s "Settling time [s]"
  Terminator : Terminator
  Terminator1 : Terminator
  Terminator2 : Terminator
  abc to Alpha-Beta-Zero : spsabctoAlphaBetaZeroLib/abc to Alpha-Beta-Zero
      settings: SourceProductBaseCode=PS
  i_d_pos : Outport
  i_q_pos : Outport  Port=2
  i_d_neg : Outport  Port=3
  i_q_neg : Outport  Port=4
  wires:
  Demux/1 -> SOGI-alpha/2(v_alpha)
  Mux1/1 -> Alpha-Beta-Zero to dq1/1
  Demux1/2 -> i_q_pos/1
  Demux/2 -> SOGI-beta/1(v_beta)
  Constant1/1 -> Mux1/3
  Mux/1 -> Alpha-Beta-Zero to dq0/1
  Constant/1 -> Mux/3
  SOGI-alpha/2(q_v_alpha_p) -> PNSC/2(q_v_alpha_p)
  abc to Alpha-Beta-Zero/1 -> Demux/1
  PNSC/3(v_alpha_neg) -> Mux1/1
  Demux/3 -> Terminator/1
  SOGI-beta/1(v_beta_p) -> PNSC/3(v_beta_p)
  Demux2/1 -> i_d_neg/1
  Demux2/2 -> i_q_neg/1
  omega/1 -> SOGI-beta/2(omega), SOGI-alpha/1(omega)
  SOGI-alpha/1(v_alpha_p) -> PNSC/1(v_alpha_p)
  PNSC/2(v_beta_pos) -> Mux/2
  PNSC/1(v_alpha_pos) -> Mux/1
  Alpha-Beta-Zero to dq0/1 -> Demux1/1
  PNSC/4(v_beta_neg) -> Mux1/2
  i_abc/1 -> abc to Alpha-Beta-Zero/1
  SOGI-beta/2(q_v_beta_p) -> PNSC/4(q_v_beta_p)
  Alpha-Beta-Zero to dq1/1 -> Demux2/1
  Demux1/3 -> Terminator1/1
  Demux2/3 -> Terminator2/1
  Demux1/1 -> i_d_pos/1
  Gain/1 -> Alpha-Beta-Zero to dq1/2
  theta_pos/1 -> Gain/1, Alpha-Beta-Zero to dq0/2

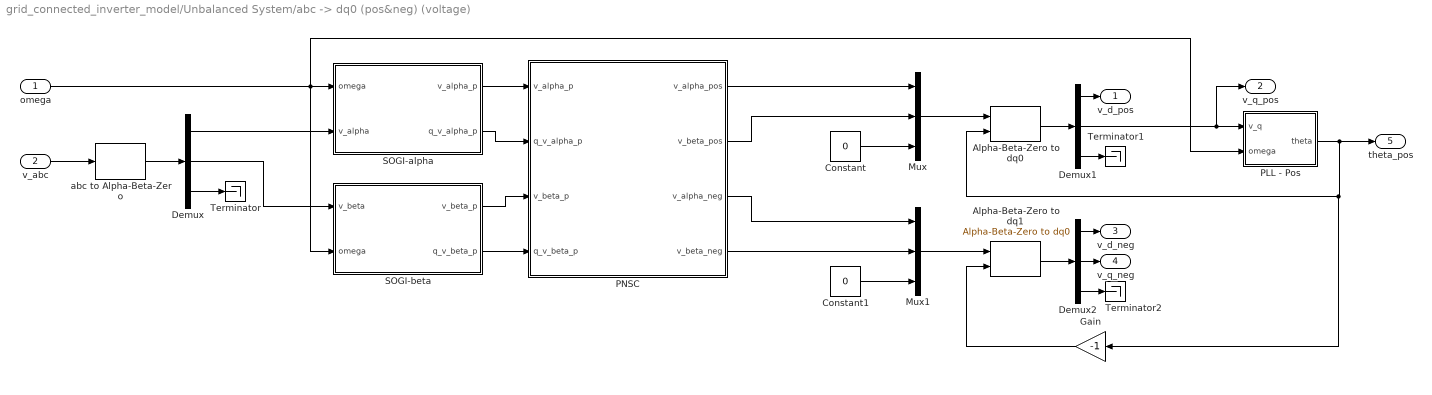
== system grid_connected_inverter_model/Unbalanced System/abc -> dq0 (pos&neg) (voltage) ==
  omega : Inport
  v_abc : Inport  Port=2
  Alpha-Beta-Zero to dq0 : spsAlphaBetaZerotodq0Lib/Alpha-Beta-Zero to dq0  Alignment=Aligned with phase A axis
      settings: SourceProductBaseCode=PS
  Alpha-Beta-Zero to dq1 : spsAlphaBetaZerotodq0Lib/Alpha-Beta-Zero to dq0  Alignment=Aligned with phase A axis
      settings: SourceProductBaseCode=PS
  Constant : Constant  Value=0
  Constant1 : Constant  Value=0
  Demux : Demux  Outputs=3
  Demux1 : Demux  Outputs=3
  Demux2 : Demux  Outputs=3
  Gain : Gain  Gain=-1
  Mux : Mux  Inputs=3
  Mux1 : Mux  Inputs=3
  PLL - Pos : Subsystem  mask{kp_mask=Kp_PLL, ki_mask=Ki_PLL}
      mask prompts: kp_mask "kp"; ki_mask "ki"
  PNSC : Subsystem
  SOGI-alpha : Subsystem  mask{t_s=0.1}
      mask prompts: t_s "Settling time [s]"
  SOGI-beta : Subsystem  mask{t_s=0.1}
      mask prompts: t_s "Settling time [s]"
  Terminator : Terminator
  Terminator1 : Terminator
  Terminator2 : Terminator
  abc to Alpha-Beta-Zero : spsabctoAlphaBetaZeroLib/abc to Alpha-Beta-Zero
      settings: SourceProductBaseCode=PS
  v_d_pos : Outport
  v_q_pos : Outport  Port=2
  v_d_neg : Outport  Port=3
  v_q_neg : Outport  Port=4
  theta_pos : Outport  Port=5
  wires:
  Demux/1 -> SOGI-alpha/2(v_alpha)
  Mux1/1 -> Alpha-Beta-Zero to dq1/1
  Demux1/2 -> v_q_pos/1, PLL - Pos/1(v_q)
  Demux/2 -> SOGI-beta/1(v_beta)
  Constant1/1 -> Mux1/3
  Mux/1 -> Alpha-Beta-Zero to dq0/1
  Constant/1 -> Mux/3
  SOGI-alpha/2(q_v_alpha_p) -> PNSC/2(q_v_alpha_p)
  abc to Alpha-Beta-Zero/1 -> Demux/1
  PNSC/3(v_alpha_neg) -> Mux1/1
  Demux/3 -> Terminator/1
  SOGI-beta/1(v_beta_p) -> PNSC/3(v_beta_p)
  Demux2/1 -> v_d_neg/1
  Demux2/2 -> v_q_neg/1
  omega/1 -> PLL - Pos/2(omega), SOGI-beta/2(omega), SOGI-alpha/1(omega)
  SOGI-alpha/1(v_alpha_p) -> PNSC/1(v_alpha_p)
  PNSC/2(v_beta_pos) -> Mux/2
  PNSC/1(v_alpha_pos) -> Mux/1
  Alpha-Beta-Zero to dq0/1 -> Demux1/1
  PNSC/4(v_beta_neg) -> Mux1/2
  v_abc/1 -> abc to Alpha-Beta-Zero/1
  SOGI-beta/2(q_v_beta_p) -> PNSC/4(q_v_beta_p)
  Alpha-Beta-Zero to dq1/1 -> Demux2/1
  Demux1/3 -> Terminator1/1
  Demux2/3 -> Terminator2/1
  PLL - Pos/1(theta) -> theta_pos/1, Gain/1, Alpha-Beta-Zero to dq0/2
  Demux1/1 -> v_d_pos/1
  Gain/1 -> Alpha-Beta-Zero to dq1/2

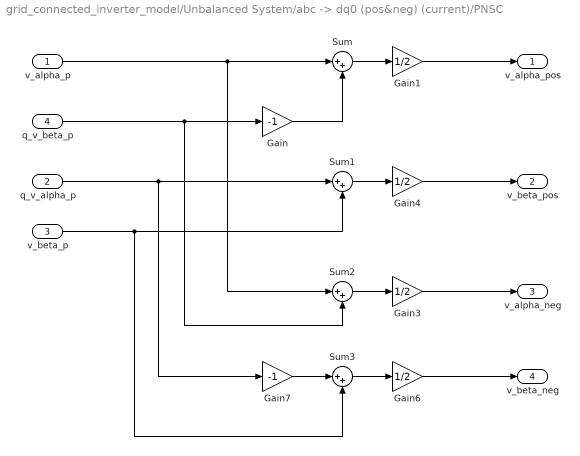
== system grid_connected_inverter_model/Unbalanced System/abc -> dq0 (pos&neg) (current)/PNSC ==
  v_alpha_p : Inport
  q_v_alpha_p : Inport  Port=2
  v_beta_p : Inport  Port=3
  q_v_beta_p : Inport  Port=4
  Gain : Gain  Gain=-1
  Gain{1,3..4,6} (4 alike) : Gain  Gain=1/2
  Gain7 : Gain  Gain=-1
  Sum{,1..3} (4 alike) : Sum  Inputs=|++
  v_alpha_pos : Outport
  v_beta_pos : Outport  Port=2
  v_alpha_neg : Outport  Port=3
  v_beta_neg : Outport  Port=4
  wires:
  Gain/1 -> Sum/2
  Sum/1 -> Gain1/1
  Sum1/1 -> Gain4/1
  q_v_beta_p/1 -> Sum2/2, Gain/1
  Sum2/1 -> Gain3/1
  v_alpha_p/1 -> Sum2/1, Sum/1
  v_beta_p/1 -> Sum3/2, Sum1/2
  Gain7/1 -> Sum3/1
  q_v_alpha_p/1 -> Sum1/1, Gain7/1
  Sum3/1 -> Gain6/1
  Gain1/1 -> v_alpha_pos/1
  Gain4/1 -> v_beta_pos/1
  Gain3/1 -> v_alpha_neg/1
  Gain6/1 -> v_beta_neg/1

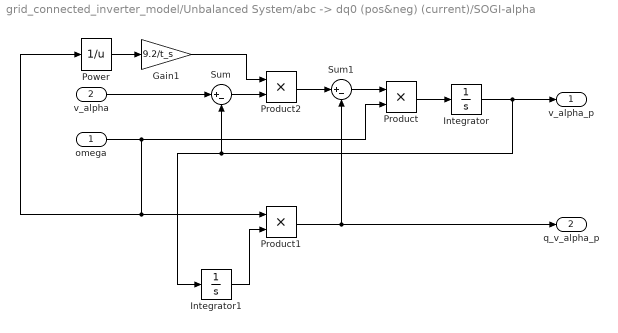
== system grid_connected_inverter_model/Unbalanced System/abc -> dq0 (pos&neg) (current)/SOGI-alpha ==
  omega : Inport
  v_alpha : Inport  Port=2
  Gain1 : Gain  Gain=9.2/t_s
  Integrator : Integrator
  Integrator1 : Integrator
  Power : Math  Operator=reciprocal  SaturateOnIntegerOverflow=on
  Product : Product
  Product1 : Product
  Product2 : Product
  Sum : Sum  Inputs=|+-
  Sum1 : Sum  Inputs=|+-
  v_alpha_p : Outport
  q_v_alpha_p : Outport  Port=2
  wires:
  v_alpha/1 -> Sum/1
  Sum/1 -> Product2/2
  Sum1/1 -> Product/1
  Product/1 -> Integrator/1
  Integrator/1 -> Integrator1/1, Sum/2, v_alpha_p/1
  omega/1 -> Power/1, Product1/1, Product/2
  Integrator1/1 -> Product1/2
  Power/1 -> Gain1/1
  Product2/1 -> Sum1/1
  Gain1/1 -> Product2/1
  Product1/1 -> q_v_alpha_p/1, Sum1/2

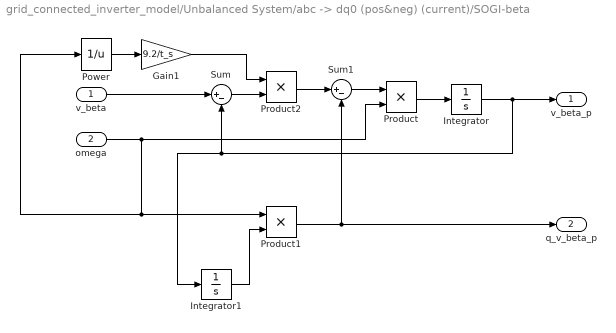
== system grid_connected_inverter_model/Unbalanced System/abc -> dq0 (pos&neg) (current)/SOGI-beta ==
  v_beta : Inport
  omega : Inport  Port=2
  Gain1 : Gain  Gain=9.2/t_s
  Integrator : Integrator
  Integrator1 : Integrator
  Power : Math  Operator=reciprocal  SaturateOnIntegerOverflow=on
  Product : Product
  Product1 : Product
  Product2 : Product
  Sum : Sum  Inputs=|+-
  Sum1 : Sum  Inputs=|+-
  v_beta_p : Outport
  q_v_beta_p : Outport  Port=2
  wires:
  v_beta/1 -> Sum/1
  Sum/1 -> Product2/2
  Sum1/1 -> Product/1
  Product/1 -> Integrator/1
  Integrator/1 -> Integrator1/1, Sum/2, v_beta_p/1
  omega/1 -> Power/1, Product1/1, Product/2
  Integrator1/1 -> Product1/2
  Power/1 -> Gain1/1
  Product2/1 -> Sum1/1
  Gain1/1 -> Product2/1
  Product1/1 -> q_v_beta_p/1, Sum1/2

== system grid_connected_inverter_model/Unbalanced System/abc -> dq0 (pos&neg) (voltage)/PLL - Pos ==
  v_q : Inport
  omega : Inport  Port=2
  Gain : Gain
  Integrator : Integrator
  PID Controller : pid_lib/PID Controller  Controller=PI  Form=Ideal  TimeDomain=Continuous-time  UseExternalTs=off  SampleTime=-1  IntegratorMethod=Forward Euler  FilterMethod=Forward Euler  ControllerParametersSource=internal  P=kp_mask  I=ki_mask  D=0  UseFilter=on  N=100  TunerSelectOption=Transfer Function Based (PID Tuner App)  InitialConditionSource=internal  InitialConditionForIntegrator=0  InitialConditionForFilter=0  DifferentiatorICPrevScaledInput=0  ExternalReset=none  TrackingMode=off  Kt=1  LimitOutput=off  SatLimitsSource=internal  UpperSaturationLimit=inf  LowerSaturationLimit=-inf  LinearizeAsGain=on  AntiWindupMode=none  Kb=1  POutMin=[]  POutMax=[]  IOutMin=[]  IOutMax=[]  DOutMin=[]  DOutMax=[]  NOutMin=[]  NOutMax=[]  SumOutMin=[]  SumOutMax=[]  SaturationOutMin=[]  SaturationOutMax=[]  PParamMin=[]  PParamMax=[]  IParamMin=[]  IParamMax=[]  DParamMin=[]  DParamMax=[]  NParamMin=[]  NParamMax=[]  KbParamMin=[]  KbParamMax=[]  KtParamMin=[]  KtParamMax=[]  KbOutMin=[]  KbOutMax=[]  KtOutMin=[]  KtOutMax=[]  IntegratorOutMin=[]  IntegratorOutMax=[]  FilterOutMin=[]  FilterOutMax=[]  SumI1OutMin=[]  SumI1OutMax=[]  SumI2OutMin=[]  SumI2OutMax=[]  SumI3OutMin=[]  SumI3OutMax=[]  SumI4OutMin=[]  SumI4OutMax=[]  SumDOutMin=[]  SumDOutMax=[]  DifferentiatorOutMin=[]  DifferentiatorOutMax=[]  FilterDiffOutCoefMin=[]  FilterDiffOutCoefMax=[]  ReciprocalOutMin=[]  ReciprocalOutMax=[]  SumDenOutMin=[]  SumDenOutMax=[]  SumNumOutMin=[]  SumNumOutMax=[]  DivideOutMin=[]  DivideOutMax=[]  UdiffTsProdOutMin=[]  UdiffTsProdOutMax=[]  NTsProdOutMin=[]  NTsProdOutMax=[]  UintegralTsProdOutMin=[]  UintegralTsProdOutMax=[]  UngainTsProdOutMin=[]  UngainTsProdOutMax=[]  IntegratorContinuousStateAttributes=''  IntegratorStateMustResolveToSignalObject=off  IntegratorRTWStateStorageClass=Auto  FilterContinuousStateAttributes=''  FilterStateMustResolveToSignalObject=off  FilterRTWStateStorageClass=Auto  ParallelPVariant=Passthrough  IdealPVariant=InternalParameters  IVariant=InternalParameters  DVariant=Disabled  IntegratorVariant=Continuous  SatVariant=Disabled  AWVariant=Passthrough  PCopyVariant=Disabled  TRVariant=Disabled  FdbkBlocksVariant=Forward  IdealPFdbkVariant=Disabled  SatFdbkVariant=Disabled  DerivativeFilterVariant=Disabled  NVariant=Disabled  NCopyVariant=Disabled_SignalSpec  FilterICVariant=Disabled  IntegratorICVariant=InternalICs  ExternalResetVariant=Disabled  TRSumVariant=Passthrough  SumFdbkVariant=Disabled  SumVariant=Sum_PI  TsampFilterVariant=InternalTs  TsampNgainVariant=Passthrough  TsampIntegralVariant=Passthrough  ExternalSaturationOutDataTypeStr=Inherit: Same as second input
  Sum : Sum  Inputs=|++
  theta : Outport
  wires:
  v_q/1 -> PID Controller/1
  omega/1 -> Sum/2
  Integrator/1 -> theta/1
  PID Controller/1 -> Sum/1
  Sum/1 -> Gain/1
  Gain/1 -> Integrator/1

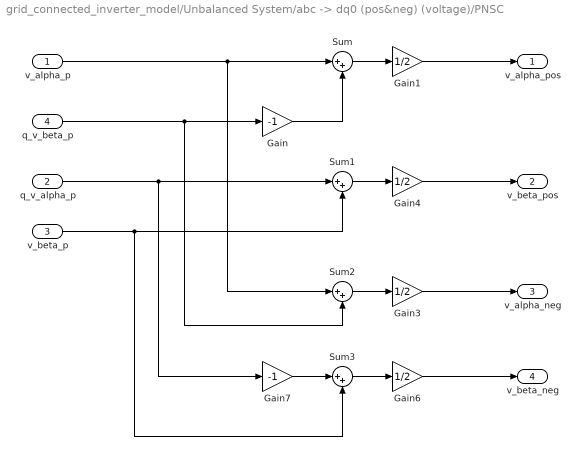
== system grid_connected_inverter_model/Unbalanced System/abc -> dq0 (pos&neg) (voltage)/PNSC ==
  v_alpha_p : Inport
  q_v_alpha_p : Inport  Port=2
  v_beta_p : Inport  Port=3
  q_v_beta_p : Inport  Port=4
  Gain : Gain  Gain=-1
  Gain{1,3..4,6} (4 alike) : Gain  Gain=1/2
  Gain7 : Gain  Gain=-1
  Sum{,1..3} (4 alike) : Sum  Inputs=|++
  v_alpha_pos : Outport
  v_beta_pos : Outport  Port=2
  v_alpha_neg : Outport  Port=3
  v_beta_neg : Outport  Port=4
  wires:
  Gain/1 -> Sum/2
  Sum/1 -> Gain1/1
  Sum1/1 -> Gain4/1
  q_v_beta_p/1 -> Sum2/2, Gain/1
  Sum2/1 -> Gain3/1
  v_alpha_p/1 -> Sum2/1, Sum/1
  v_beta_p/1 -> Sum3/2, Sum1/2
  Gain7/1 -> Sum3/1
  q_v_alpha_p/1 -> Sum1/1, Gain7/1
  Sum3/1 -> Gain6/1
  Gain1/1 -> v_alpha_pos/1
  Gain4/1 -> v_beta_pos/1
  Gain3/1 -> v_alpha_neg/1
  Gain6/1 -> v_beta_neg/1

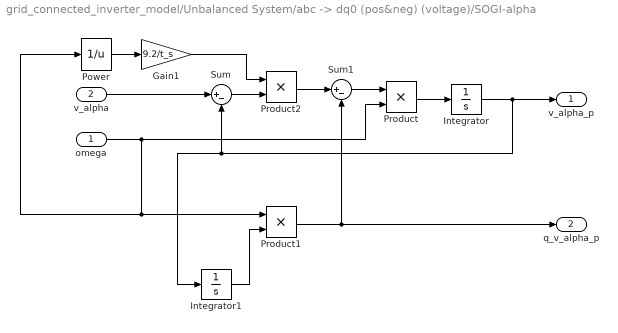
== system grid_connected_inverter_model/Unbalanced System/abc -> dq0 (pos&neg) (voltage)/SOGI-alpha ==
  omega : Inport
  v_alpha : Inport  Port=2
  Gain1 : Gain  Gain=9.2/t_s
  Integrator : Integrator
  Integrator1 : Integrator
  Power : Math  Operator=reciprocal  SaturateOnIntegerOverflow=on
  Product : Product
  Product1 : Product
  Product2 : Product
  Sum : Sum  Inputs=|+-
  Sum1 : Sum  Inputs=|+-
  v_alpha_p : Outport
  q_v_alpha_p : Outport  Port=2
  wires:
  v_alpha/1 -> Sum/1
  Sum/1 -> Product2/2
  Sum1/1 -> Product/1
  Product/1 -> Integrator/1
  Integrator/1 -> Integrator1/1, Sum/2, v_alpha_p/1
  omega/1 -> Power/1, Product1/1, Product/2
  Integrator1/1 -> Product1/2
  Power/1 -> Gain1/1
  Product2/1 -> Sum1/1
  Gain1/1 -> Product2/1
  Product1/1 -> q_v_alpha_p/1, Sum1/2

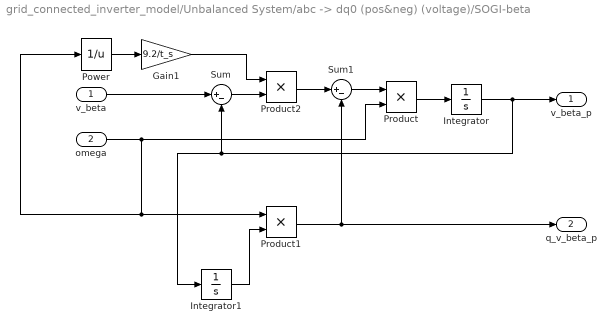
== system grid_connected_inverter_model/Unbalanced System/abc -> dq0 (pos&neg) (voltage)/SOGI-beta ==
  v_beta : Inport
  omega : Inport  Port=2
  Gain1 : Gain  Gain=9.2/t_s
  Integrator : Integrator
  Integrator1 : Integrator
  Power : Math  Operator=reciprocal  SaturateOnIntegerOverflow=on
  Product : Product
  Product1 : Product
  Product2 : Product
  Sum : Sum  Inputs=|+-
  Sum1 : Sum  Inputs=|+-
  v_beta_p : Outport
  q_v_beta_p : Outport  Port=2
  wires:
  v_beta/1 -> Sum/1
  Sum/1 -> Product2/2
  Sum1/1 -> Product/1
  Product/1 -> Integrator/1
  Integrator/1 -> Integrator1/1, Sum/2, v_beta_p/1
  omega/1 -> Power/1, Product1/1, Product/2
  Integrator1/1 -> Product1/2
  Power/1 -> Gain1/1
  Product2/1 -> Sum1/1
  Gain1/1 -> Product2/1
  Product1/1 -> q_v_beta_p/1, Sum1/2
